simulink model "Torres22210429"  (R2023a)
settings: Solver=ode15s  StartTime=0.0  StopTime=30.0  MaxStep=1E-3  RelTol=1e-3
libraries: slpidlib x1
settings Model: LastModifiedBy=diegt
settings DataIOCC: ReturnWorkspaceOutputs=off  TimeSaveName=t
settings DebuggingCC: AlgebraicLoopMsg=none  ArtificialAlgebraicLoopMsg=none  MaxConsecutiveZCsMsg=none  ModelReferenceExtraNoncontSigs=none  OperatingPointInterfaceChecksumMismatchMsg=none
settings RTWCC: GPUComputeCapability=5.0

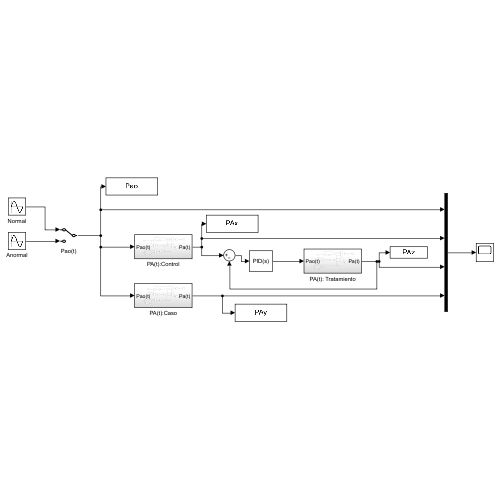
[thumbnail: Simulink's stored preview of the top-level diagram]
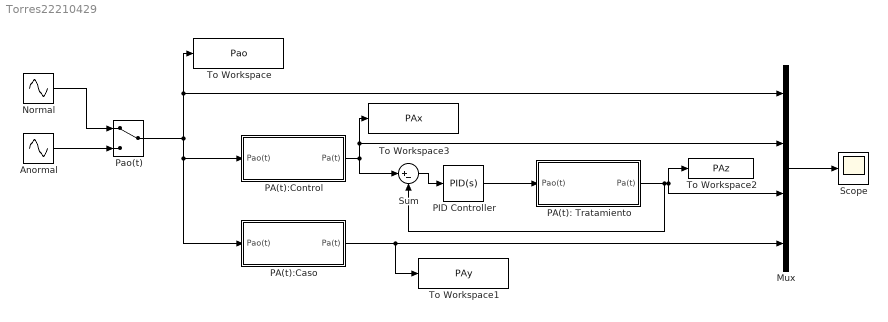
== system Torres22210429 ==
  Anormal : Sin  Amplitude=1.5  Frequency=pi  SampleTime=0
  Mux : Mux
  Normal : Sin  Amplitude=2.5  Frequency=pi/2  SampleTime=0
  PA(t): Tratamiento : Subsystem
  PA(t):Caso : Subsystem
  PA(t):Control : Subsystem
  PID Controller : slpidlib/PID Controller  Controller=PID  Form=Parallel  TimeDomain=Continuous-time  UseExternalTs=off  SampleTime=-1  IntegratorMethod=Forward Euler  FilterMethod=Forward Euler  ControllerParametersSource=internal  P=2092.696  I=33557.427  UseKiTs=off  D=10.009  N=228565.595208321  UseFilter=on  TunerSelectOption=Transfer Function Based (PID Tuner App)  InitialConditionSource=internal  InitialConditionForIntegrator=0  InitialConditionForFilter=0  DifferentiatorICPrevScaledInput=0  ExternalReset=none  TrackingMode=off  Kt=1  LimitOutput=off  SatLimitsSource=internal  UpperSaturationLimit=inf  LowerSaturationLimit=-inf  LinearizeAsGain=on  AntiWindupMode=none  Kb=1  LimitIntegrator=off  UpperIntegratorSaturationLimit=inf  LowerIntegratorSaturationLimit=-inf  POutMin=[]  POutMax=[]  IOutMin=[]  IOutMax=[]  DOutMin=[]  DOutMax=[]  NOutMin=[]  NOutMax=[]  SumOutMin=[]  SumOutMax=[]  SaturationOutMin=[]  SaturationOutMax=[]  PParamMin=[]  PParamMax=[]  IParamMin=[]  IParamMax=[]  DParamMin=[]  DParamMax=[]  NParamMin=[]  NParamMax=[]  KbParamMin=[]  KbParamMax=[]  KtParamMin=[]  KtParamMax=[]  KbOutMin=[]  KbOutMax=[]  KtOutMin=[]  KtOutMax=[]  IntegratorOutMin=[]  IntegratorOutMax=[]  FilterOutMin=[]  FilterOutMax=[]  SumI1OutMin=[]  SumI1OutMax=[]  SumI2OutMin=[]  SumI2OutMax=[]  SumI3OutMin=[]  SumI3OutMax=[]  SumI4OutMin=[]  SumI4OutMax=[]  SumDOutMin=[]  SumDOutMax=[]  DifferentiatorOutMin=[]  DifferentiatorOutMax=[]  FilterDiffOutCoefMin=[]  FilterDiffOutCoefMax=[]  ReciprocalOutMin=[]  ReciprocalOutMax=[]  SumDenOutMin=[]  SumDenOutMax=[]  SumNumOutMin=[]  SumNumOutMax=[]  DivideOutMin=[]  DivideOutMax=[]  UdiffTsProdOutMin=[]  UdiffTsProdOutMax=[]  NTsProdOutMin=[]  NTsProdOutMax=[]  UintegralTsProdOutMin=[]  UintegralTsProdOutMax=[]  UngainTsProdOutMin=[]  UngainTsProdOutMax=[]  ClampingZeroOutDataTypeStr=Inherit: Inherit via back propagation  ClampingZeroOutMin=[]  ClampingZeroOutMax=[]  FilterDenConstantOutDataTypeStr=Inherit: Inherit via back propagation  FilterDenConstantOutMin=[]  FilterDenConstantOutMax=[]  PCopyOutDataTypeStr=Inherit: Inherit via back propagation  PCopyOutMin=[]  PCopyOutMax=[]  NCopyOutDataTypeStr=Inherit: Inherit via back propagation  NCopyOutMin=[]  NCopyOutMax=[]  IntegratorContinuousStateAttributes=''  IntegratorStateMustResolveToSignalObject=off  IntegratorRTWStateStorageClass=Auto  FilterContinuousStateAttributes=''  FilterStateMustResolveToSignalObject=off  FilterRTWStateStorageClass=Auto  ParallelPVariant=InternalParameters  IdealPVariant=Disabled  IVariant=InternalParameters  DVariant=InternalParameters  IntegratorVariant=Continuous  SatVariant=Disabled  AWVariant=Passthrough  PCopyVariant=Disabled  TRVariant=Disabled  FdbkBlocksVariant=Forward  IdealPFdbkVariant=Disabled  SatFdbkVariant=Disabled  DerivativeFilterVariant=ContFilter  NVariant=InternalParameters  NCopyVariant=Disabled  FilterICVariant=InternalICsFilter  IntegratorICVariant=InternalICs  ExternalResetVariant=Disabled  TRSumVariant=Passthrough  SumFdbkVariant=Disabled  SumVariant=Sum_PID  TsampFilterVariant=InternalTs  TsampNgainVariant=Passthrough  TsampIntegralVariant=Disabled_SignalSpec  ExternalSaturationOutDataTypeStr=Inherit: Same as second input
  Pao(t) : ManualSwitch
  Scope : Scope
  Sum : Sum  Inputs=|+-
  To Workspace : ToWorkspace  VariableName=Pao  SampleTime=-1
  To Workspace1 : ToWorkspace  VariableName=PAy  SampleTime=-1
  To Workspace2 : ToWorkspace  VariableName=PAz  SampleTime=-1
  To Workspace3 : ToWorkspace  VariableName=PAx  SampleTime=-1
  wires:
  Mux/1 -> Scope/1
  Pao(t)/1 -> PA(t):Control/1(Pao(t)), PA(t):Caso/1(Pao(t)), Mux/1, To Workspace/1
  Anormal/1 -> Pao(t)/2
  Normal/1 -> Pao(t)/1
  PA(t):Control/1(Pa(t)) -> Mux/2, To Workspace3/1, Sum/1
  PA(t):Caso/1(Pa(t)) -> To Workspace1/1, Mux/4
  PA(t): Tratamiento/1(Pa(t)) -> Sum/2, Mux/3, To Workspace2/1
  Sum/1 -> PID Controller/1
  PID Controller/1 -> PA(t): Tratamiento/1(Pao(t))

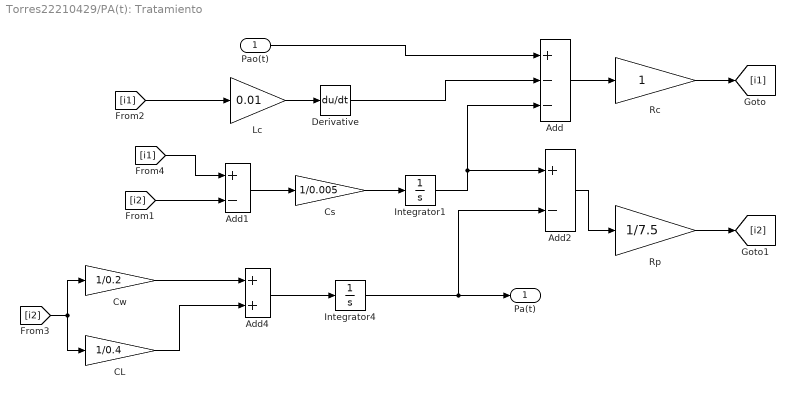
== system Torres22210429/PA(t): Tratamiento ==
  Pao(t) : Inport
  Add : Sum  Inputs=+--
  Add1 : Sum  Inputs=+-
  Add2 : Sum  Inputs=+-
  Add4 : Sum
  CL : Gain  Gain=1/0.4
  Cs : Gain  Gain=1/0.005
  Cw : Gain  Gain=1/0.2
  Derivative : Derivative
  Integrator1 : Integrator
  Integrator4 : Integrator
  Lc : Gain  Gain=0.01
  Rc : Gain
  Rp : Gain  Gain=1/7.5
  Pa(t) : Outport
  wires:
  [i1] -> Add1/1
  CL/1 -> Add4/2
  Add/1 -> Rc/1
  Pao(t)/1 -> Add/1
  Integrator4/1 -> Add2/2, Pa(t)/1
  Integrator1/1 -> Add2/1, Add/3
  Rc/1 -> [i1]
  Add4/1 -> Integrator4/1
  [i1] -> Lc/1
  [i2] -> Add1/2
  Derivative/1 -> Add/2
  Lc/1 -> Derivative/1
  Cs/1 -> Integrator1/1
  Add1/1 -> Cs/1
  Cw/1 -> Add4/1
  [i2] -> CL/1, Cw/1
  Rp/1 -> [i2]
  Add2/1 -> Rp/1

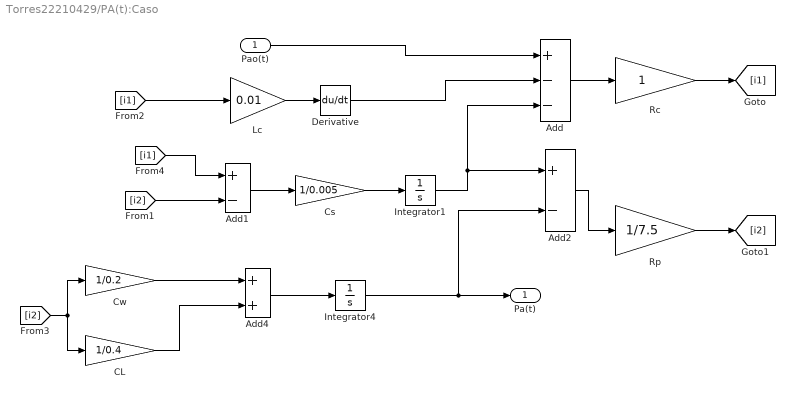
== system Torres22210429/PA(t):Caso ==
  Pao(t) : Inport
  Add : Sum  Inputs=+--
  Add1 : Sum  Inputs=+-
  Add2 : Sum  Inputs=+-
  Add4 : Sum
  CL : Gain  Gain=1/0.4
  Cs : Gain  Gain=1/0.005
  Cw : Gain  Gain=1/0.2
  Derivative : Derivative
  Integrator1 : Integrator
  Integrator4 : Integrator
  Lc : Gain  Gain=0.01
  Rc : Gain
  Rp : Gain  Gain=1/7.5
  Pa(t) : Outport
  wires:
  Cw/1 -> Add4/1
  [i2] -> CL/1, Cw/1
  Add1/1 -> Cs/1
  Integrator1/1 -> Add2/1, Add/3
  Add4/1 -> Integrator4/1
  Integrator4/1 -> Add2/2, Pa(t)/1
  Lc/1 -> Derivative/1
  Derivative/1 -> Add/2
  Rp/1 -> [i2]
  Cs/1 -> Integrator1/1
  Rc/1 -> [i1]
  [i2] -> Add1/2
  Pao(t)/1 -> Add/1
  [i1] -> Lc/1
  CL/1 -> Add4/2
  Add/1 -> Rc/1
  Add2/1 -> Rp/1
  [i1] -> Add1/1

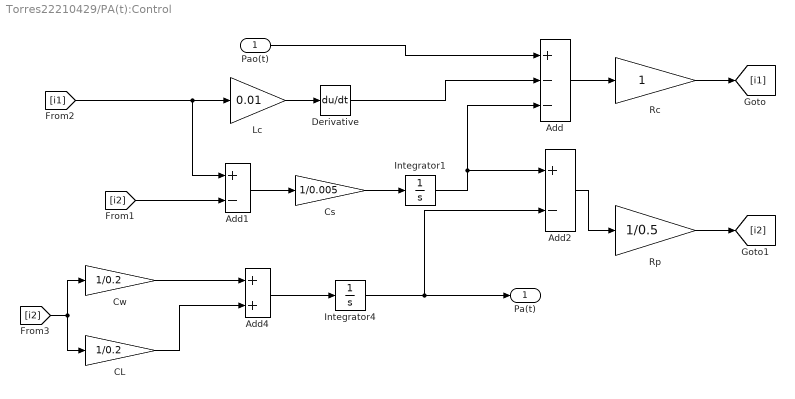
== system Torres22210429/PA(t):Control ==
  Pao(t) : Inport
  Add : Sum  Inputs=+--
  Add1 : Sum  Inputs=+-
  Add2 : Sum  Inputs=+-
  Add4 : Sum
  CL : Gain  Gain=1/0.2
  Cs : Gain  Gain=1/0.005
  Cw : Gain  Gain=1/0.2
  Derivative : Derivative
  Integrator1 : Integrator
  Integrator4 : Integrator
  Lc : Gain  Gain=0.01
  Rc : Gain
  Rp : Gain  Gain=1/0.5
  Pa(t) : Outport
  wires:
  Add/1 -> Rc/1
  Rp/1 -> [i2]
  Rc/1 -> [i1]
  Add2/1 -> Rp/1
  Lc/1 -> Derivative/1
  Derivative/1 -> Add/2
  [i1] -> Add1/1, Lc/1
  Cs/1 -> Integrator1/1
  Integrator1/1 -> Add2/1, Add/3
  Add1/1 -> Cs/1
  [i2] -> Add1/2
  Cw/1 -> Add4/1
  CL/1 -> Add4/2
  [i2] -> CL/1, Cw/1
  Add4/1 -> Integrator4/1
  Integrator4/1 -> Add2/2, Pa(t)/1
  Pao(t)/1 -> Add/1
